simulink model "TV_2017old"  (R2016a)
settings: Solver=FixedStepAuto  StartTime=0.0  StopTime=inf  FixedStep=0.001  RelTol=1e-3
PreLoadFcn:
  | TV_2017_parameters
values from neighbouring files (symbols this model uses):
  battery_voltage = single(530)    [HIL_parameters.m]    (also in HIL_parameters_2018.m; TV_2017_parameters.m; TV_2017_parameters_VD.m)
  car_params = Simulink_Car_params    [HIL_parameters.m]    (also in HIL_parameters_2018.m; TV_2017_parameters.m; TV_2017_parameters_VD.m)
  i_Diff = 16    [HIL_parameters.m]    (also in HIL_parameters_2018.m; TV_2017_parameters.m)
  Kp = 1    [HIL_parameters.m]    (also in HIL_parameters_2018.m; TV_2017_parameters.m; TV_2017_parameters_VD.m)
  motor_data = struct    [HIL_parameters.m]    (also in HIL_parameters_2018.m; TV_2017_parameters.m)
  powerLimitControl = Simulink_el    [HIL_parameters.m]    (also in HIL_parameters_2018.m; TV_2017_parameters.m; TV_2017_parameters_VD.m)
  settings = Simulink_Settings    [HIL_parameters.m]    (also in HIL_parameters_2018.m; TV_2017_parameters.m; TV_2017_parameters_VD.m)
  SpdC_BCC = 0    [HIL_parameters.m]    (also in HIL_parameters_2018.m; TV_2017_parameters.m; TV_2017_parameters_VD.m)
  Speed_Neg_sat = -21    [HIL_parameters.m]    (also in HIL_parameters_2018.m; TV_2017_parameters.m; TV_2017_parameters_VD.m)
  Speed_Pos_sat = 21    [HIL_parameters.m]    (also in HIL_parameters_2018.m; TV_2017_parameters.m; TV_2017_parameters_VD.m)
  SteeringAngleFL = [-23.80 -22.65 -21.50 -20.34 -19.18 -18.03 -16.86 -15.70 -14.53 -13.35 -12.18 -10.99 -9.80 -8.61 -7.40 -6.19 -4.97 -3.75 -2.51 -1.26 0 1.27 2.56 3.85 5.17 6.50 7.84 9.21 10.59 12.00 13.42 14.88 16.36 17.87 19.41 20.99 22.61 24.26 25.97 27.73 29.54]    [CarSetupAnalysis2018.m]    (also in HIL_parameters_2018.m; TV_2017_parameters.m; TV_2017_parameters_VD.m = [-24.129 -22.950 -21.772 -20.593 -19.413 -18.232 -17.050 -15)
  SteeringAngleFR = [-29.54 -27.73 -25.97 -24.26 -22.61 -20.99 -19.41 -17.87 -16.36 -14.88 -13.42 -12.00 -10.59 -9.21 -7.84 -6.50 -5.17 -3.85 -2.56 -1.27 0 1.26 2.51 3.75 4.97 6.19 7.40 8.61 9.80 10.99 12.18 13.35 14.53 15.70 16.86 18.03 19.18 20.34 21.50 22.65 23.80]    [CarSetupAnalysis2018.m]    (also in HIL_parameters_2018.m; TV_2017_parameters.m; TV_2017_parameters_VD.m = [-29.3050 -27.5340 -25.8140 -24.1410 -22.5110 -20.9180 -19.3)
  SteeringWhAngle = [-105 -99.75 -94.5 -89.25 -84 -78.75 -73.5 -68.25 -63 -57.75 -52.5 -47.25 -42 -36.75 -31.5 -26.25 -21.0 -15.75 -10.5 -5.25 0.0 5.25 10.50 15.75 21.00 26.25 31.50 36.75 42.00 47.25 52.50 57.75  63.00 68.25 73.50 78.75 84.00 89.25 94.50 99.75 105.00]    [TV_2017_parameters_VD.m]
  Tn_n = 0    [HIL_parameters.m]    (also in HIL_parameters_2018.m; TV_2017_parameters.m; TV_2017_parameters_VD.m)
  tractionControl = Simulink_tc    [HIL_parameters.m]    (also in HIL_parameters_2018.m; IterativeTractionControlTuning.m; TV_2017_parameters.m; TV_2017_parameters_VD.m)
  yawRateControl = Simulink_yawRate    [HIL_parameters.m]    (also in HIL_parameters_2018.m; TV_2017_parameters.m; TV_2017_parameters_VD.m)
undefined symbols (not defined in the file or in its folder): DiscIntNeverNeededParam, magnitude, speedEstimation, TC_Decr_Gas, TC_Derivative, TC_Incr_Gas, TC_On, TC_Relay_Off, TC_Relay_On
libraries: CarMaker4SL x274, simulink_extras x45, simulink x37, dspfdesign x2
(part 2 of 14)

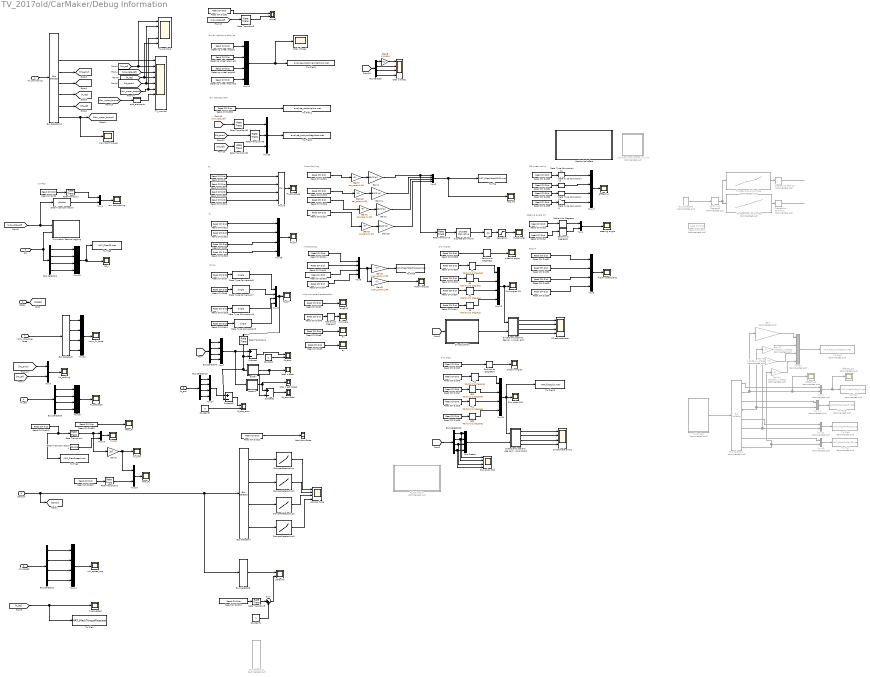
== system TV_2017old/CarMaker/Debug Information  ==
  note: SimRes
  note: Eff wheel radius
  note: motortorques
  note: Friction
  note: FZ CM
  note: Fy
  note: FX
  note: misc movement acceleration
  note: Steering angle CM
  note: Motor Rpm log
  note: Slip Angles
  note: Slip rates
  note: Yaw rate regulator
  note: Driver intentions analyze
  TV_monitoring : Inport
  states : Inport  Port=2
  whl_speed : Inport  Port=3
  Fx_est : Inport  Port=4
  "SR " : Inport  Port=5
  Sensors : Inport  Port=6
  norm_long_tire_force : Inport  Port=7
  Fz_acc : Inport  Port=8
  Abs : Abs
  "Aero downforce " : Scope
  Aero_Fx : Scope
  Aero_Fz : Scope
  Bus Creator : BusCreator  Inputs=4
  Bus Selector : BusSelector  OutputSignals=power,Input_throttle,Input_brake,KERS_pos
  Bus Selector1 : BusSelector  Commented=on  OutputSignals=Pm_FL,Pe_FL,Pm_FR,Pe_FR,Pm_RL,Pe_RL,Pm_RR,Pe_RR
  Bus Selector10 : BusSelector  OutputSignals=SR_FL,SR_FR,SR_RL,SR_RR
  Bus Selector11 : BusSelector  Commented=on  OutputSignals=steering_wheel_angle
  Bus Selector12 : BusSelector  OutputSignals=active_contraints,saturated_constraints,percentage_delivered_torque,Mz_error,yaw_rate_ref,T_req,Mz_ref,maxMotorTorque
  Bus Selector{2..5,13} (5 alike) : BusSelector  OutputSignals=FL,FR,RL,RR
  Bus Selector6 : BusSelector  OutputSignals=Fz_FL,Fz_FR,Fz_RL,Fz_RR
  Bus Selector7 : BusSelector  OutputSignals=damper_rate_FL,damper_rate_FR,damper_rate_RL,damper_rate_RR
  Bus Selector8 : BusSelector  OutputSignals=steering_wheel_angle
  Bus Selector9 : BusSelector  Commented=on  OutputSignals=steering_wheel_angle
  Constant : Constant  Value=0
  Constant1 : Constant
  Constant2 : Constant  Value=0
  DamperRateLookup : Lookup_n-D  NumberOfTableDimensions=1  BreakpointsForDimension1=car_params.damper_table_breakpoint;  Table=car_params.damper_pull_push_values_front;  ExtrapMethod=Clip  UseLastTableValue=on  InternalRulePriority=Speed  RndMeth=Simplest  InputSameDT=on
  DamperRateLookup1 : Lookup_n-D  NumberOfTableDimensions=1  BreakpointsForDimension1=car_params.damper_table_breakpoint;  Table=car_params.damper_pull_push_values_front;  ExtrapMethod=Clip  UseLastTableValue=on  InternalRulePriority=Speed  RndMeth=Simplest  InputSameDT=on
  DamperRateLookup2 : Lookup_n-D  NumberOfTableDimensions=1  BreakpointsForDimension1=car_params.damper_table_breakpoint;  Table=car_params.damper_pull_push_values_rear;  ExtrapMethod=Clip  UseLastTableValue=on  InternalRulePriority=Speed  RndMeth=Simplest  InputSameDT=on
  DamperRateLookup3 : Lookup_n-D  NumberOfTableDimensions=1  BreakpointsForDimension1=car_params.damper_table_breakpoint;  Table=car_params.damper_pull_push_values_rear;  ExtrapMethod=Clip  UseLastTableValue=on  InternalRulePriority=Speed  RndMeth=Simplest  InputSameDT=on
  Data Type Conversion : DataTypeConversion  OutDataTypeStr=double
  Data Type Conversion1 : DataTypeConversion  OutDataTypeStr=double
  Data Type Conversion{6..13} (8 alike) : DataTypeConversion  OutDataTypeStr=single
  Degrees to Radians : simulink_extras/Transformations/Degrees to Radians  Commented=on
  Degrees to Radians1 : simulink_extras/Transformations/Degrees to Radians  Commented=on
  Discrete Derivative : simulink/Discrete/Discrete Derivative  gainval=1.0  ICPrevScaledInput=0.0  InputProcessing=Inherited  OutMin=[]  OutMax=[]  OutDataType=fixdt(1, 16)  OutScaling=2^-10  DoSatur=off
  Extract and scale to deg compare to CM output in individual error : Subsystem
  Extract and scale to deg compare to CM output in individual error1 : Subsystem
  FL : simulink_extras/Transformations/Radians to Degrees
  FL steer ang lookup deg : Lookup_n-D  Commented=on  NumberOfTableDimensions=1  BreakpointsForDimension1=SteeringWhAngle  Table=SteeringAngleFL  ExtrapMethod=Clip  UseLastTableValue=on  InternalRulePriority=Speed  RndMeth=Simplest  InputSameDT=on
  FL1 : simulink_extras/Transformations/Radians to Degrees
  FR : simulink_extras/Transformations/Radians to Degrees
  FR steer ang lookup deg : Lookup_n-D  Commented=on  NumberOfTableDimensions=1  BreakpointsForDimension1=SteeringWhAngle  Table=SteeringAngleFR  ExtrapMethod=Clip  UseLastTableValue=on  InternalRulePriority=Speed  RndMeth=Simplest  InputSameDT=on
  FR1 : simulink_extras/Transformations/Radians to Degrees
  FY_CM : Scope
  Fl_derivate : Scope
  Fx_CM_scope : Scope
  Fx_estScope : Scope
  Fz_CM : Scope
  Fz_Estimation : Subsystem  Commented=on  TreatAsAtomicUnit=on
  Fz_acc_error : Scope  NumInputPorts=2
  Fz_error : Scope  NumInputPorts=2
  Fz_error total : Scope
  Gain{,12..14} (4 alike) : Gain  Commented=on  Gain=1/battery_voltage
  Gain{1,3,7,10} (4 alike) : Gain  Gain=car_params.GR
  Gain{2,4,11,15} (4 alike) : Gain  Gain=60/(2*pi)
  Gain5 : Gain  Gain=1/car_params.GR
  Gain6 : Gain  Gain=1/car_params.GR
  Gain8 : Gain  Gain=1/10000
  Gain9 : Gain  Gain=3.6
  Mechanical effect : Subsystem
  "Motor Torques " : Scope
  Mux{1,4,9..10,20} (5 alike) : Mux  Inputs=2
  Mux{5,11..13} (4 alike) : Mux  Commented=on  Inputs=2
  Mux{2..3,6..8,14..19,22..24,26..27} (16 alike) : Mux
  Mux21 : Mux  Commented=on
  Mux25 : Mux  Inputs=3
  Mz_tracking : Scope
  RL : simulink_extras/Transformations/Radians to Degrees
  RL1 : simulink_extras/Transformations/Radians to Degrees
  RR : simulink_extras/Transformations/Radians to Degrees
  RR1 : simulink_extras/Transformations/Radians to Degrees
  Radians to Degrees{,1..2,4,7} (5 alike) : simulink_extras/Transformations/Radians to Degrees
  Radians to Degrees3 : simulink_extras/Transformations/Radians to Degrees  Commented=on
  Rate Transition{,1..5} (6 alike) : RateTransition  OutPortSampleTime=matlab_params.control_system_sample_time
  Rate Transition{6,49..51} (4 alike) : RateTransition  OutPortSampleTimeOpt=Inherit
  Read CM Dict : CarMaker4SL/Read CM Dict  xname=Vhcl.FL.Fx  xsync=off
  Read CM Dict1 : CarMaker4SL/Read CM Dict  xname=Car.LongSlipRL  xsync=off
  Read CM Dict10 : CarMaker4SL/Read CM Dict  xname=Car.vx  xsync=off
  Read CM Dict11 : CarMaker4SL/Read CM Dict  xname=Vhcl.RR.Fz  xsync=off
  Read CM Dict12 : CarMaker4SL/Read CM Dict  xname=Car.Aero.Frc_1.z  xsync=off
  Read CM Dict13 : CarMaker4SL/Read CM Dict  xname=Vhcl.Steer.Ang  xsync=off
  Read CM Dict14 : CarMaker4SL/Read CM Dict  Commented=on  xsync=off
  Read CM Dict15 : CarMaker4SL/Read CM Dict  xname=Car.LongSlipRR  xsync=off
  Read CM Dict16 : CarMaker4SL/Read CM Dict  xname=Car.LongSlipRL  xsync=off
  Read CM Dict17 : CarMaker4SL/Read CM Dict  xname=Car.SlipAngleRR  xsync=off
  Read CM Dict18 : CarMaker4SL/Read CM Dict  xname=Vhcl.FR.Fx  xsync=off
  Read CM Dict19 : CarMaker4SL/Read CM Dict  xname=Vhcl.RR.Fx  xsync=off
  Read CM Dict2 : CarMaker4SL/Read CM Dict  xname=Car.YawRate  xsync=off
  Read CM Dict20 : CarMaker4SL/Read CM Dict  xname=Vhcl.RL.Fx  xsync=off
  Read CM Dict21 : CarMaker4SL/Read CM Dict  xname=Vhcl.FL.Fy  xsync=off
  Read CM Dict22 : CarMaker4SL/Read CM Dict  xname=Vhcl.FR.Fy  xsync=off
  Read CM Dict23 : CarMaker4SL/Read CM Dict  xname=Vhcl.RR.Fy  xsync=off
  Read CM Dict24 : CarMaker4SL/Read CM Dict  xname=Car.WheelSpd_FL  xsync=off
  Read CM Dict25 : CarMaker4SL/Read CM Dict  xname=Car.WheelSpd_FR  xsync=off
  Read CM Dict26 : CarMaker4SL/Read CM Dict  xname=Car.WheelSpd_RL  xsync=off
  Read CM Dict27 : CarMaker4SL/Read CM Dict  xname=Car.WheelSpd_RR  xsync=off
  Read CM Dict28 : CarMaker4SL/Read CM Dict  xname=Vhcl.RL.Fz  xsync=off
  Read CM Dict29 : CarMaker4SL/Read CM Dict  xname=Car.muRoadRL  xsync=off
  Read CM Dict3 : CarMaker4SL/Read CM Dict  xname=Car.CFR.rz  xsync=off
  Read CM Dict30 : CarMaker4SL/Read CM Dict  xname=Car.muRoadRR  xsync=off
  Read CM Dict31 : CarMaker4SL/Read CM Dict  xname=Car.muRoadFL  xsync=off
  Read CM Dict32 : CarMaker4SL/Read CM Dict  xname=Car.muRoadFR  xsync=off
  Read CM Dict33 : CarMaker4SL/Read CM Dict  xname=Car.WFL.Radius  xsync=off
  Read CM Dict34 : CarMaker4SL/Read CM Dict  xname=Car.WFR.Radius  xsync=off
  Read CM Dict35 : CarMaker4SL/Read CM Dict  xname=Car.WRR.Radius  xsync=off
  Read CM Dict36 : CarMaker4SL/Read CM Dict  xname=Car.WRL.Radius  xsync=off
  Read CM Dict37 : CarMaker4SL/Read CM Dict  xname=Car.SlipAngleRL  xsync=off
  Read CM Dict38 : CarMaker4SL/Read CM Dict  xname=Car.SideSlipAngle  xsync=off
  Read CM Dict39 : CarMaker4SL/Read CM Dict  xname=Car.SlipAngleFL  xsync=off
  Read CM Dict4 : CarMaker4SL/Read CM Dict  xname=Car.CFL.rz  xsync=off
  Read CM Dict40 : CarMaker4SL/Read CM Dict  xname=Car.SlipAngleFR  xsync=off
  Read CM Dict41 : CarMaker4SL/Read CM Dict  xname=PT.WFL.Trq_Drive  xsync=off
  Read CM Dict42 : CarMaker4SL/Read CM Dict  xname=PT.WFR.Trq_Drive  xsync=off
  Read CM Dict43 : CarMaker4SL/Read CM Dict  xname=PT.WRL.Trq_Drive  xsync=off
  Read CM Dict44 : CarMaker4SL/Read CM Dict  xname=PT.WRR.Trq_Drive  xsync=off
  Read CM Dict45 : CarMaker4SL/Read CM Dict  xname=Car.SideSlipAngle  xsync=off
  Read CM Dict46 : CarMaker4SL/Read CM Dict  xname=Car.LongSlipFL  xsync=off
  Read CM Dict47 : CarMaker4SL/Read CM Dict  xname=Car.LongSlipFR  xsync=off
  Read CM Dict48 : CarMaker4SL/Read CM Dict  xname=Vhcl.Roll  xsync=off
  Read CM Dict49 : CarMaker4SL/Read CM Dict  xname=Car.Aero.Frc_1.z  xsync=off
  Read CM Dict5 : CarMaker4SL/Read CM Dict  xname=Vhcl.RL.Fy  xsync=off
  Read CM Dict50 : CarMaker4SL/Read CM Dict  xname=Vhcl.YawRate  xsync=off
  Read CM Dict51 : CarMaker4SL/Read CM Dict  xname=Vhcl.YawRate  xsync=off
  Read CM Dict53 : CarMaker4SL/Read CM Dict  xname=Car.Aero.Frc_1.x  xsync=off
  Read CM Dict6 : CarMaker4SL/Read CM Dict  xname=Vhcl.FR.Fz  xsync=off
  Read CM Dict7 : CarMaker4SL/Read CM Dict  xname=Vhcl.FL.Fz  xsync=off
  Read CM Dict8 : CarMaker4SL/Read CM Dict  xname=Car.ax  xsync=off
  Read CM Dict9 : CarMaker4SL/Read CM Dict  xname=Car.ay  xsync=off
  SA calculation : Subsystem
  SA estimate error : Scope  NumInputPorts=4
  SA estimate error1 : Scope  NumInputPorts=4
  SR_i : Scope
  Saturation : Saturate  UpperLimit=50000
  Simulation Results Logging : Subsystem
  Slip angles CM : Scope
  Slip ratios CM1 : Scope
  Slip ratios CM2 : Scope  NumInputPorts=4
  Steering wheel ang-vel2 : CarMaker4SL/Read CM Dict  xname=DM.Steer.AngVel  xsync=off
  Steering wheel ang-vel3 : CarMaker4SL/Read CM Dict  xname=DM.Brake  xsync=off
  Steering wheel angle2 : CarMaker4SL/Read CM Dict  xname=DM.Steer.Ang  xsync=off
  Steering wheel angle3 : CarMaker4SL/Read CM Dict  xname=DM.Gas  xsync=off
  Subsystem : Subsystem  Commented=on
  Subtract : Sum  Inputs=+-
  Subtract1 : Sum  Inputs=+-
  Subtract2 : Sum  Inputs=+-
  Sum : Sum  Inputs=|++
  TV_monitor : Scope  NumInputPorts=9
  TV_monitor1 : Scope  NumInputPorts=5
  "T_requested " : Scope
  To File : ToFile  Filename=MAT_files\MotorRPMS.mat  MatrixName=MotorRpms  SaveFormat=Timeseries
  To File1 : ToFile  Filename=MAT_files\TorqueRequest  MatrixName=TorqueRequest  SaveFormat=Timeseries
  To File10 : ToFile  Filename=analyse_mat/yawRegulator.mat  MatrixName=yaw_reg  SaveFormat=Timeseries
  To File11 : ToFile  Filename=analyse_mat/trueYaw.mat  MatrixName=vhclYaw  SaveFormat=Timeseries
  To File12 : ToFile  Filename=analyse_mat/driverIntentions.mat  MatrixName=driverIntentions  SaveFormat=Timeseries
  To File13 : ToFile  Filename=MAT_files\slip.mat  MatrixName=slipratio  SaveFormat=Timeseries
  To File2 : ToFile  Filename=MAT_files\Speed.mat  MatrixName=VehicleSpeed  SaveFormat=Timeseries
  To File3 : ToFile  Filename=MAT_files\MotorTorques.mat  MatrixName=MotorTorques  SaveFormat=Timeseries
  To File4 : ToFile  Commented=on  Filename=MAT_files\PmPe_FL.mat  MatrixName=PmPe_FL  SaveFormat=Timeseries
  To File5 : ToFile  Commented=on  Filename=MAT_files\PmPe_FR.mat  MatrixName=PmPe_FR  SaveFormat=Timeseries
  To File6 : ToFile  Commented=on  Filename=MAT_files\PmPe_RL.mat  MatrixName=PmPe_RL  SaveFormat=Timeseries
  To File7 : ToFile  Commented=on  Filename=MAT_files\PmPe_RR.mat  MatrixName=PmPe_RR  SaveFormat=Timeseries
  To File8 : ToFile  Filename=MAT_files\SR.mat  MatrixName=SR  SaveFormat=Timeseries
  To File9 : ToFile  Commented=on  Filename=MAT_files\currentDraw.mat  SaveFormat=Timeseries
  Vehicle dynamics analysis JMH : Subsystem  Commented=on
  Vx_kmh : Scope
  "Vx_ms " : Scope
  Yaw rate tracking : Scope
  add_elements : Subsystem
  addall : Subsystem
  addall1 : Subsystem
  ax : Scope
  ay : Scope
  damper force : Scope  NumInputPorts=4
  delta SW : Scope  NumInputPorts=2
  effRadius : Scope
  effectFL_el : Scope  Commented=on
  effectFL_el1 : Scope  Commented=on
  eng rot : Scope
  friction coefficients : Scope
  "longSlip " : Scope
  maxMotorTorques : Scope
  norm_Fx_force : Scope
  rollAngle : Scope
  sideslip angle : Scope
  sideslip angle1 : Scope
  steering angle : Scope
  total z estimated : Scope
  total z force : Scope
  total z force1 : Scope
  total z force2 : Scope  NumInputPorts=4
  whl_speed_cog : Scope
  yawref : Scope  NumInputPorts=2
  wires:
  [T_req] -> To File1/1, "T_requested "/1
  [Mz_error] -> Mux9/1  "error"
  [Mz_ref] -> Mux9/2  "ref"
  Mux9/1 -> Mz_tracking/1
  Mux5/1 -> effectFL_el1/1, To File4/1
  Mux11/1 -> To File5/1
  Mux12/1 -> To File6/1
  Mux13/1 -> To File7/1
  Subsystem/1(Power debug) -> Bus Selector1/1
  Bus Selector1/1 -> Mux5/1  "<Pm_FL>"
  Bus Selector1/2 -> Gain/1, effectFL_el/1, Mux5/2  "<Pe_FL>"
  Bus Selector1/3 -> Mux11/1  "<Pm_FR>"
  Bus Selector1/4 -> Gain12/1, Mux11/2  "<Pe_FR>"
  Bus Selector1/5 -> Mux12/1  "<Pm_RL>"
  Bus Selector1/6 -> Gain13/1, Mux12/2  "<Pe_RL>"
  Bus Selector1/7 -> Mux13/1  "<Pm_RR>"
  Bus Selector1/8 -> Gain14/1, Mux13/2  "<Pe_RR>"
  whl_speed/1 -> Bus Selector2/1
  Bus Selector2/4 -> Mux14/4  "<RR>"
  Bus Selector2/3 -> Mux14/3  "<RL>"
  Bus Selector2/2 -> Mux14/2  "<FR>"
  Bus Selector2/1 -> Mux14/1  "<FL>"
  Mux14/1 -> whl_speed_cog/1
  Fx_est/1 -> Bus Selector3/1
  Bus Selector3/1 -> Mux15/1  "<FL>"
  Bus Selector3/2 -> Mux15/2  "<FR>"
  Bus Selector3/3 -> Mux15/3  "<RL>"
  Bus Selector3/4 -> Mux15/4  "<RR>"
  Mux15/1 -> Fx_estScope/1
  Read CM Dict53/1 -> Aero_Fx/1  "FL"
  Read CM Dict10/1 -> To File2/1, Rate Transition1/1  "V_x"
  Mux10/1 -> "Vx_ms "/1
  Rate Transition1/1 -> Gain9/1, Mux10/1  "V_x"
  Data Type Conversion1/1 -> Mux10/2  "V_est"
  Gain9/1 -> Mux20/1, Vx_kmh/1
  Mux20/1 -> Aero_Fz/1
  Read CM Dict49/1 -> Rate Transition2/1  "FL"
  Rate Transition2/1 -> Mux20/2
  Gain/1 -> Mux21/1  "Current FL"
  Gain12/1 -> Mux21/2  "Current FR"
  Gain13/1 -> Mux21/3  "Current RL"
  Gain14/1 -> Mux21/4  "Current RR"
  Mux21/1 -> To File9/1
  norm_long_tire_force/1 -> Bus Selector5/1
  Bus Selector5/1 -> Mux22/1  "<FL>"
  Bus Selector5/4 -> Mux22/4  "<RR>"
  Bus Selector5/3 -> Mux22/3  "<RL>"
  Bus Selector5/2 -> Mux22/2  "<FR>"
  Mux22/1 -> norm_Fx_force/1
  Rate Transition3/1 -> Discrete Derivative/1
  Saturation/1 -> Fl_derivate/1
  Abs/1 -> Saturation/1
  Discrete Derivative/1 -> Abs/1
  Mux2/1 -> eng rot/1, To File/1
  Read CM Dict27/1 -> Gain3/1
  Read CM Dict26/1 -> Gain1/1
  Gain15/1 -> Mux2/4  "Motor_RPM"
  Gain3/1 -> Gain15/1
  Gain2/1 -> Mux2/3  "Motor_RPM"
  Gain1/1 -> Gain2/1
  Gain11/1 -> Mux2/2  "Motor_RPM"
  Gain10/1 -> Gain11/1
  Read CM Dict25/1 -> Gain10/1
  Read CM Dict24/1 -> Gain7/1
  Gain4/1 -> Mux2/1, Rate Transition3/1  "Motor_RPM"
  Gain7/1 -> Gain4/1
  Radians to Degrees1/1 -> Mux4/2
  Mux4/1 -> steering angle/1
  Read CM Dict3/1 -> Radians to Degrees/1
  Read CM Dict4/1 -> Radians to Degrees1/1
  Radians to Degrees/1 -> Mux4/1
  Read CM Dict48/1 -> Radians to Degrees7/1
  Radians to Degrees7/1 -> rollAngle/1
  Read CM Dict9/1 -> ay/1
  Read CM Dict8/1 -> ax/1
  Read CM Dict1/1 -> "longSlip "/1
  Mux16/1 -> Fx_CM_scope/1
  Read CM Dict18/1 -> Mux16/2  "Fx_FR"
  Read CM Dict19/1 -> Mux16/4  "Fx_RR"
  Read CM Dict20/1 -> Mux16/3  "Fx_RL"
  Read CM Dict/1 -> Mux16/1  "Fx_FL"
  Mux18/1 -> FY_CM/1
  Read CM Dict22/1 -> Mux18/2  "Fy_FR"
  Read CM Dict5/1 -> Mux18/3  "Fy_RL"
  Read CM Dict23/1 -> Mux18/4  "Fy_RR"
  Read CM Dict21/1 -> Mux18/1  "Fy_FL"
  Data Type Conversion10/1 -> Mux3/3  "RL"
  Data Type Conversion7/1 -> Mux3/2  "FR"
  Mux3/1 -> Rate Transition4/1, Fz_CM/1
  Read CM Dict7/1 -> Data Type Conversion8/1
  Read CM Dict11/1 -> Data Type Conversion9/1
  Read CM Dict6/1 -> Data Type Conversion7/1
  Data Type Conversion9/1 -> Mux3/4  "RR"
  Read CM Dict28/1 -> Data Type Conversion10/1
  Data Type Conversion8/1 -> Mux3/1  "FL"
  Read CM Dict30/1 -> Mux6/4  "RR"
  Read CM Dict29/1 -> Mux6/3  "RL"
  Read CM Dict32/1 -> Mux6/2  "FR"
  Mux6/1 -> friction coefficients/1
  Read CM Dict31/1 -> Mux6/1  "FL"
  Gain6/1 -> To File3/1
  Gain5/1 -> "Motor Torques "/1
  Read CM Dict43/1 -> Mux8/3  "Mot_RL"
  Read CM Dict44/1 -> Mux8/4  "Mot_RR"
  Read CM Dict41/1 -> Mux8/1  "Mot_FL"
  Mux8/1 -> Gain6/1, Gain5/1
  Read CM Dict42/1 -> Mux8/2  "Mot_FR"
  Mux17/1 -> effRadius/1
  Data Type Conversion6/1 -> Mux17/4  "R_RR"
  Read CM Dict35/1 -> Data Type Conversion6/1
  Read CM Dict34/1 -> Data Type Conversion13/1
  Data Type Conversion13/1 -> Mux17/2  "R_FR"
  Data Type Conversion11/1 -> Mux17/3  "R_RL"
  Data Type Conversion12/1 -> Mux17/1  "R_FL"
  Read CM Dict36/1 -> Data Type Conversion11/1
  Read CM Dict33/1 -> Data Type Conversion12/1
  Read CM Dict38/1 -> Radians to Degrees2/1
  Radians to Degrees2/1 -> sideslip angle/1
  Mux23/1 -> Extract and scale to deg compare to CM output in individual error/1(SA_CM), Slip angles CM/1
  Read CM Dict40/1 -> FR/1  "FR"
  Read CM Dict39/1 -> FL/1  "FL"
  Read CM Dict17/1 -> RR/1  "RL"
  RR/1 -> Mux23/4
  Read CM Dict37/1 -> RL/1  "RL"
  RL/1 -> Mux23/3
  FR/1 -> Mux23/2
  FL/1 -> Mux23/1
  [yaw_rate_ref] -> Data Type Conversion/1, Simulation Results Logging/1(r_ref)  "r_ref"
  Bus Selector4/4 -> Mux19/4  "<RR>"
  Mux19/1 -> SR_i/1, To File8/1
  Bus Selector4/1 -> Mux19/1  "<FL>"
  Bus Selector4/2 -> Mux19/2  "<FR>"
  Bus Selector4/3 -> Mux19/3  "<RL>"
  "SR "/1 -> Simulation Results Logging/2(SR), Bus Selector4/1
  Data Type Conversion/1 -> Mux1/2  "r_ref"
  Rate Transition/1 -> Mux1/1  "r"
  Mux1/1 -> Yaw rate tracking/1
  Read CM Dict2/1 -> Rate Transition/1  "r"
  Subtract/1 -> Fz_error/1
  Bus Selector6/1 -> Mux7/1  "<Fz_FL>"
  Bus Selector6/2 -> Mux7/2  "<Fz_FR>"
  Bus Selector6/3 -> Mux7/3  "<Fz_RL>"
  Bus Selector6/4 -> Mux7/4  "<Fz_RR>"
  Mux7/1 -> addall1/1(In1), Subtract/1
  Rate Transition4/1 -> Subtract2/2, addall/1(In1), Subtract/2
  addall/1(Out1) -> Subtract1/2, total z force/1
  addall1/1(Out1) -> total z estimated/1, Subtract1/1
  Subtract1/1 -> Fz_error total/1
  Read CM Dict12/1 -> "Aero downforce "/1
  DamperRateLookup/1 -> damper force/1  "Fz_damp_FL"
  Bus Selector7/1 -> DamperRateLookup/1  "<damper_rate_FL>"
  Bus Selector7/2 -> DamperRateLookup1/1  "<damper_rate_FR>"
  Bus Selector7/3 -> DamperRateLookup2/1  "<damper_rate_RL>"
  Bus Selector7/4 -> DamperRateLookup3/1  "<damper_rate_RR>"
  DamperRateLookup1/1 -> damper force/2
  DamperRateLookup2/1 -> damper force/3
  DamperRateLookup3/1 -> damper force/4
  Sensors/1 -> [sensor], Bus Selector8/1, Bus Selector7/1  "V_est"
  Constant/1 -> Fz_error/2
  Bus Selector8/1 -> delta SW/1  "<steering_wheel_angle>"
  Read CM Dict13/1 -> Rate Transition5/1
  Rate Transition5/1 -> Sum/1
  Sum/1 -> delta SW/2
  Constant1/1 -> Sum/2
  [states] -> Bus Selector6/1
  states/1 -> [states]
  SA calculation/1(Out1) -> Extract and scale to deg compare to CM output in individual error/2(In1)
  [sensor] -> SA calculation/1(In1)
  Extract and scale to deg compare to CM output in individual error/1(FL) -> SA estimate error/1
  Extract and scale to deg compare to CM output in individual error/2(FR) -> SA estimate error/2
  Extract and scale to deg compare to CM output in individual error/3(RL) -> SA estimate error/3
  Extract and scale to deg compare to CM output in individual error/4(RR) -> SA estimate error/4
  Radians to Degrees3/1 -> FL steer ang lookup deg/1, FR steer ang lookup deg/1
  Degrees to Radians1/1 -> ?
  FR steer ang lookup deg/1 -> Degrees to Radians1/1
  Degrees to Radians/1 -> ?
  FL steer ang lookup deg/1 -> Degrees to Radians/1
  Bus Selector9/1 -> Radians to Degrees3/1  "<steering_wheel_angle>"
  Read CM Dict45/1 -> Radians to Degrees4/1
  Radians to Degrees4/1 -> sideslip angle1/1
  Mux24/1 -> Extract and scale to deg compare to CM output in individual error1/1(SA_CM), To File13/1, Slip ratios CM1/1
  Read CM Dict47/1 -> FR1/1  "FR"
  Read CM Dict46/1 -> FL1/1  "FL"
  Read CM Dict15/1 -> RR1/1  "RL"
  RR1/1 -> Mux24/4
  Read CM Dict16/1 -> RL1/1  "RL"
  RL1/1 -> Mux24/3
  FR1/1 -> Mux24/2
  FL1/1 -> Mux24/1
  Extract and scale to deg compare to CM output in individual error1/1(FL) -> SA estimate error1/1
  Extract and scale to deg compare to CM output in individual error1/2(FR) -> SA estimate error1/2
  Extract and scale to deg compare to CM output in individual error1/3(RL) -> SA estimate error1/3
  Extract and scale to deg compare to CM output in individual error1/4(RR) -> SA estimate error1/4
  Bus Selector10/1 -> Slip ratios CM2/1, Bus Creator/1  "<SR_FL>"
  Bus Selector10/2 -> Slip ratios CM2/2, Bus Creator/2  "<SR_FR>"
  Bus Selector10/3 -> Slip ratios CM2/3, Bus Creator/3  "<SR_RL>"
  Bus Selector10/4 -> Slip ratios CM2/4, Bus Creator/4  "<SR_RR>"
  [states] -> Bus Selector10/1
  Bus Creator/1 -> Extract and scale to deg compare to CM output in individual error1/2(In1)
  TV_monitoring/1 -> Bus Selector12/1
  Bus Selector12/3 -> TV_monitor/1  "<percentage_delivered_torque>"
  Bus Selector12/4 -> [Mz_error]  "<Mz_error>"
  Bus Selector12/5 -> [yaw_rate_ref]  "<yaw_rate_ref>"
  Bus Selector12/6 -> [T_req]  "<T_req>"
  Bus Selector12/7 -> [Mz_ref]  "<Mz_ref>"
  [Mz_ref] -> TV_monitor1/1, TV_monitor/2
  [yaw_rate_ref] -> TV_monitor/3
  [T_req] -> TV_monitor1/5, TV_monitor/4
  [Mz_error] -> TV_monitor1/2, TV_monitor/5
  Read CM Dict50/1 -> To File11/1
  Rate Transition50/1 -> Mux25/1
  Rate Transition49/1 -> Mux25/2
  Rate Transition51/1 -> Mux25/3
  [yaw_rate_ref] -> Rate Transition50/1
  [Mz_error] -> Rate Transition49/1
  [Mz_ref] -> Rate Transition51/1
  Mux25/1 -> To File10/1
  Steering wheel ang-vel2/1 -> Mux26/2
  Steering wheel angle3/1 -> Mux26/3
  Steering wheel ang-vel3/1 -> Mux26/4
  Steering wheel angle2/1 -> Mux26/1
  Mux26/1 -> total z force1/1, To File12/1
  Bus Selector12/8 -> maxMotorTorques/1, [Max_motor_torque]  "<maxMotorTorque>"
  [Max_motor_torque] -> TV_monitor1/4, TV_monitor/6
  [Max_motor_torque] -> add_elements/1(In1)
  add_elements/1(Out1) -> TV_monitor/7
  ? -> Bus Selector11/1
  [states] -> Bus Selector/1
  Bus Selector/1 -> Gain8/1  "<power>"
  Bus Selector/2 -> total z force2/2  "<Input_throttle>"
  Bus Selector/3 -> total z force2/3  "<Input_brake>"
  Bus Selector/4 -> total z force2/4  "<KERS_pos>"
  Gain8/1 -> total z force2/1
  Read CM Dict51/1 -> yawref/1
  [yaw_rate_ref] -> Rate Transition6/1
  Rate Transition6/1 -> yawref/2
  Constant2/1 -> Fz_acc_error/2
  Subtract2/1 -> Fz_acc_error/1
  Bus Selector13/1 -> Mux27/1  "<FL>"
  Bus Selector13/2 -> Mux27/2  "<FR>"
  Bus Selector13/3 -> Mux27/3  "<RL>"
  Bus Selector13/4 -> Mux27/4  "<RR>"
  Fz_acc/1 -> Bus Selector13/1
  Mux27/1 -> Subtract2/1

== system TV_2017old/CarMaker/DrivMan3 ==
  note: There's rarely a reason to override DrivMan signals.
      | Use the VehicleControl interface for this purpose.
  Sync_In : Inport
  Env.Misc : Inport  Port=2
  BusCreator : BusCreator  Inputs=17
  Demux : Demux  Outputs=17
  DrivMan : S-Function  FunctionName=CM_Sfun  Parameters='DrivMan'  SFunctionDeploymentMode=off  EnableBusSupport=off
  Sync_Out : Outport
  DrivMan.Out : Outport  Port=2
  wires:
  Demux/17 -> BusCreator/17  "DrivMan Steering Trq"
  Demux/16 -> BusCreator/16  "DrivMan Steering AngAcc"
  Demux/15 -> BusCreator/15  "DrivMan Steering AngVel"
  Demux/14 -> BusCreator/14  "DrivMan Steering Ang"
  Demux/13 -> BusCreator/13  "DrivMan Gas"
  Demux/12 -> BusCreator/12  "DrivMan Clutch"
  Demux/11 -> BusCreator/11  "DrivMan BrakePark"
  Demux/10 -> BusCreator/10  "DrivMan Brake"
  Demux/9 -> BusCreator/9  "DrivMan GearNo"
  Demux/8 -> BusCreator/8  "DrivMan SelectorCtrl"
  Demux/7 -> BusCreator/7  "DrivMan UserSignal4"
  Demux/6 -> BusCreator/6  "DrivMan UserSignal3"
  Demux/5 -> BusCreator/5  "DrivMan UserSignal2"
  Demux/4 -> BusCreator/4  "DrivMan UserSignal1"
  Demux/3 -> BusCreator/3  "DrivMan UserSignal0"
  Demux/2 -> BusCreator/2  "DrivMan Key"
  Demux/1 -> BusCreator/1  "DrivMan SST"
  Env.Misc/1 -> DrivMan/2
  Sync_In/1 -> DrivMan/1
  DrivMan/1 -> Sync_Out/1
  BusCreator/1 -> DrivMan.Out/1
  DrivMan/2 -> Demux/1

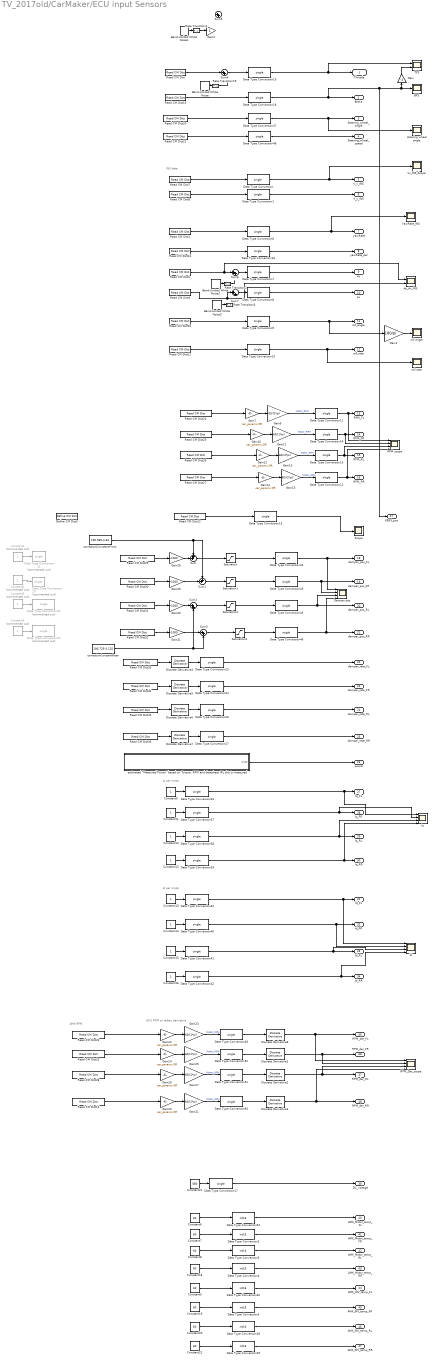
== system TV_2017old/CarMaker/ECU input Sensors  ==
  note: INS data
  note: ECU RPM to radian derivative
  note: AMK RPM
  note: Id per motor
  note: Iq per motor
  Ay_Ax_INS : Scope  NumInputPorts=2
  BPS : Scope
  Band-Limited White Noise : simulink/Sources/Band-Limited White Noise  Cov=[0.00002]  Ts=0.1  seed=[23341]
  Band-Limited White Noise1 : simulink/Sources/Band-Limited White Noise  Cov=[0.00002]  Ts=0.1  seed=[23341]
  Band-Limited White Noise2 : simulink/Sources/Band-Limited White Noise  Cov=[0.01]  Ts=0.1  seed=[23341]
  Band-Limited White Noise3 : simulink/Sources/Band-Limited White Noise  Cov=[0.01]  Ts=0.1  seed=[23341]
  Constant{1..4} (4 alike) : Constant  Commented=on
  Constant{9..16} (8 alike) : Constant
  Constant{5..8,18..20,22} (8 alike) : Constant  Value=60
  Constant21 : Constant  Value=580
  Damper pos : Scope  NumInputPorts=4
  Data Type Conversion{,1,6..19,24..27,32..33,37..52} (38 alike) : DataTypeConversion  OutDataTypeStr=single
  Data Type Conversion{2..5,28..30,54} (8 alike) : DataTypeConversion  OutDataTypeStr=int16
  Data Type Conversion{20..23} (4 alike) : DataTypeConversion  Commented=on  OutDataTypeStr=single
  Define CM Dict3 : CarMaker4SL/Define CM Dict  xname=KERS_pos  xmono=off  xtype=Double  xdvaplace=None  xnstates=0  xfirststate=0  xinitial=0
  Discrete Derivative{1..3,8} (4 alike) : simulink/Discrete/Discrete Derivative  gainval=1.0  ICPrevScaledInput=0.0  InputProcessing=Inherited  OutMin=[]  OutMax=[]  OutDataType=fixdt(1, 16)  OutScaling=2^-10  DoSatur=off
  Discrete Derivative{4..7} (4 alike) : simulink/Discrete/Discrete Derivative  gainval=1.0  ICPrevScaledInput=0.0  OutMin=[]  OutMax=[]  OutDataType=fixdt(1, 16)  OutScaling=2^-10  DoSatur=off
  Gain : Gain  Gain=-1
  Gain1 : Gain  Gain=180/pi
  Gain{7,10,12,14,20,22,24,26} (8 alike) : Gain  Gain=car_params.GR
  Gain{9,11,13,15,21,23,25,27} (8 alike) : Gain  Gain=60/(2*pi)
  Gain2 : Gain
  Gain{28..31} (4 alike) : Gain  Gain=-1000
  Id : Scope  NumInputPorts=4
  Iq : Scope  NumInputPorts=4
  RPM scope : Scope  NumInputPorts=4
  "RPM_Der_scope " : Scope  NumInputPorts=4
  Rate Transition{1..3,19} (4 alike) : RateTransition  OutPortSampleTimeOpt=Inherit  OutPortSampleTime=matlab_params.sensor_sampling_time
  Read CM Dict : CarMaker4SL/Read CM Dict  xname=VC.Gas  xsync=off
  Read CM Dict1 : CarMaker4SL/Read CM Dict  xname=Vhcl.YawRate  xsync=off
  Read CM Dict10 : CarMaker4SL/Read CM Dict  xname=Vhcl.Roll  xsync=off
  Read CM Dict11 : CarMaker4SL/Read CM Dict  xname=Vhcl.RollVel  xsync=off
  Read CM Dict12 : CarMaker4SL/Read CM Dict  xname=KERS_pos  xsync=off
  Read CM Dict13 : CarMaker4SL/Read CM Dict  xname=Vhcl.YawAcc  xsync=off
  Read CM Dict14 : CarMaker4SL/Read CM Dict  xname=Car.WheelSpd_RR  xsync=off
  Read CM Dict15 : CarMaker4SL/Read CM Dict  xname=VC.Brake  xsync=off
  Read CM Dict2 : CarMaker4SL/Read CM Dict  xname=Car.ay  xsync=off
  Read CM Dict20 : CarMaker4SL/Read CM Dict  xname=Vhcl.Steer.Ang  xsync=off
  Read CM Dict21 : CarMaker4SL/Read CM Dict  xname=Vhcl.Steer.Vel  xsync=off
  Read CM Dict22 : CarMaker4SL/Read CM Dict  xname=Car.WheelSpd_FL  xsync=off
  Read CM Dict23 : CarMaker4SL/Read CM Dict  xname=Car.WheelSpd_FR  xsync=off
  Read CM Dict24 : CarMaker4SL/Read CM Dict  xname=Car.WheelSpd_FL  xsync=off
  Read CM Dict25 : CarMaker4SL/Read CM Dict  xname=Car.WheelSpd_FR  xsync=off
  Read CM Dict26 : CarMaker4SL/Read CM Dict  xname=Car.WheelSpd_RL  xsync=off
  Read CM Dict27 : CarMaker4SL/Read CM Dict  xname=Car.WheelSpd_RR  xsync=off
  Read CM Dict28 : CarMaker4SL/Read CM Dict  xname=Car.WheelSpd_RL  xsync=off
  Read CM Dict29 : CarMaker4SL/Read CM Dict  xname=Car.SpringFL.l  xsync=off
  Read CM Dict30 : CarMaker4SL/Read CM Dict  xname=Car.SpringFR.l  xsync=off
  Read CM Dict31 : CarMaker4SL/Read CM Dict  xname=Car.SpringRL.l  xsync=off
  Read CM Dict32 : CarMaker4SL/Read CM Dict  xname=Car.SpringRR.l  xsync=off
  Read CM Dict33 : CarMaker4SL/Read CM Dict  xname=Car.SpringFL.l  xsync=off
  Read CM Dict34 : CarMaker4SL/Read CM Dict  xname=Car.SpringFR.l  xsync=off
  Read CM Dict35 : CarMaker4SL/Read CM Dict  xname=Car.SpringRL.l  xsync=off
  Read CM Dict36 : CarMaker4SL/Read CM Dict  xname=Car.SpringRR.l  xsync=off
  Read CM Dict7 : CarMaker4SL/Read CM Dict  xname=Car.vx  xsync=off
  Read CM Dict8 : CarMaker4SL/Read CM Dict  xname=Car.vy  xsync=off
  Read CM Dict9 : CarMaker4SL/Read CM Dict  xname=Car.ax  xsync=off
  Saturation{,1..3} (4 alike) : Saturate  UpperLimit=200  LowerLimit=0.001
  Scope : Scope
  Sum : Sum  Inputs=++|
  Sum1 : Sum  Inputs=++|
  Sum{2..7} (6 alike) : Sum  Inputs=|++
  TPS : Scope  NumInputPorts=2
  Vx_INS_Scope : Scope
  YawRate_INS : Scope
  correctionConstantRear : Constant  Value=190.725-3.125
  correctionCornstantFront : Constant  Value=190.965-3.63
  "estimated \"Measured Power\" based on Torque, RPM and datasheet IRL this is measured" : Subsystem
  "roll angle " : Scope
  roll rate : Scope
  steering wheel angle : Scope
  "Throttle " : Outport
  "Brake " : Outport  Port=2
  "Steering_wheel_angle " : Outport  Port=3
  Steering_wheel_speed : Outport  Port=4
  V_x_INS : Outport  Port=5
  V_y_INS : Outport  Port=6
  yawRate : Outport  Port=7
  yawRate_der : Outport  Port=8
  ay : Outport  Port=9
  "ax " : Outport  Port=10
  roll_angle : Outport  Port=11
  roll_rate : Outport  Port=12
  RPM_FL : Outport  Port=13
  RPM_FR : Outport  Port=14
  RPM_RL : Outport  Port=15
  RPM_RR : Outport  Port=16
  KERS_pos : Outport  Port=17
  damper_pos_FL : Outport  Port=18
  damper_pos_FR : Outport  Port=19
  damper_pos_RL : Outport  Port=20
  damper_pos_RR : Outport  Port=21
  damper_rate_FL : Outport  Port=22
  damper_rate_FR : Outport  Port=23
  damper_rate_RL : Outport  Port=24
  damper_rate_RR : Outport  Port=25
  power : Outport  Port=26
  Iq_FL : Outport  Port=27
  Iq_FR : Outport  Port=28
  Iq_RL : Outport  Port=29
  Iq_RR : Outport  Port=30
  Id_FL : Outport  Port=31
  Id_FR : Outport  Port=32
  Id_RL : Outport  Port=33
  Id_RR : Outport  Port=34
  RPM_der_FL : Outport  Port=35
  RPM_der_FR : Outport  Port=36
  RPM_der_RL : Outport  Port=37
  RPM_der_RR : Outport  Port=38
  DC_voltage : Outport  Port=39
  AMK_Motor_temp_FL : Outport  Port=40
  AMK_Motor_temp_FR : Outport  Port=41
  AMK_Motor_temp_RL : Outport  Port=42
  AMK_Motor_temp_RR : Outport  Port=43
  AMK_INV_temp_FL : Outport  Port=44
  AMK_INV_temp_FR : Outport  Port=45
  AMK_INV_temp_RL : Outport  Port=46
  AMK_INV_temp_RR : Outport  Port=47
  wires:
  Gain7/1 -> Gain9/1
  Read CM Dict24/1 -> Gain7/1
  Read CM Dict25/1 -> Gain10/1
  Gain10/1 -> Gain11/1
  Gain12/1 -> Gain13/1
  Gain14/1 -> Gain15/1
  Read CM Dict26/1 -> Gain12/1
  Read CM Dict27/1 -> Gain14/1
  Gain9/1 -> Data Type Conversion11/1  "Motor_RPM"
  Gain15/1 -> Data Type Conversion12/1  "Motor_RPM"
  Gain13/1 -> Data Type Conversion13/1  "Motor_RPM"
  Gain11/1 -> Data Type Conversion14/1  "Motor_RPM"
  Data Type Conversion11/1 -> RPM scope/1, RPM_FL/1
  Data Type Conversion14/1 -> RPM scope/2, RPM_FR/1
  Data Type Conversion13/1 -> RPM scope/3, RPM_RL/1
  Data Type Conversion12/1 -> RPM scope/4, RPM_RR/1
  Read CM Dict12/1 -> Data Type Conversion15/1
  Data Type Conversion15/1 -> Scope/1
  Read CM Dict15/1 -> Data Type Conversion18/1
  Data Type Conversion18/1 -> KERS_pos/1, BPS/1, Gain/1, "Brake "/1
  Data Type Conversion19/1 -> TPS/1, "Throttle "/1
  Constant1/1 -> Data Type Conversion21/1
  Constant2/1 -> Data Type Conversion20/1
  Constant3/1 -> Data Type Conversion22/1
  Constant4/1 -> Data Type Conversion23/1
  Data Type Conversion25/1 -> damper_rate_FL/1
  Discrete Derivative4/1 -> Data Type Conversion25/1
  Data Type Conversion24/1 -> damper_rate_FR/1
  Discrete Derivative5/1 -> Data Type Conversion24/1
  Data Type Conversion26/1 -> damper_rate_RL/1
  Discrete Derivative6/1 -> Data Type Conversion26/1
  Data Type Conversion27/1 -> damper_rate_RR/1
  Discrete Derivative7/1 -> Data Type Conversion27/1
  Read CM Dict20/1 -> Data Type Conversion47/1
  Read CM Dict21/1 -> Data Type Conversion48/1
  Data Type Conversion47/1 -> steering wheel angle/1, "Steering_wheel_angle "/1
  Data Type Conversion48/1 -> Steering_wheel_speed/1
  Data Type Conversion17/1 -> DC_voltage/1
  Constant21/1 -> Data Type Conversion17/1
  Read CM Dict30/1 -> Gain29/1
  Read CM Dict31/1 -> Gain30/1
  Read CM Dict32/1 -> Gain31/1
  Read CM Dict29/1 -> Gain28/1
  Data Type Conversion43/1 -> Damper pos/2, damper_pos_FR/1
  Data Type Conversion45/1 -> Damper pos/3, damper_pos_RL/1
  Data Type Conversion44/1 -> Damper pos/1, damper_pos_FL/1
  Data Type Conversion46/1 -> Damper pos/4, damper_pos_RR/1
  Sum/1 -> Saturation/1
  Gain30/1 -> Sum2/1
  Gain31/1 -> Sum3/1
  correctionConstantRear/1 -> Sum3/2, Sum2/2
  Sum1/1 -> Saturation1/1
  Sum2/1 -> Saturation2/1
  Sum3/1 -> Saturation3/1
  Saturation/1 -> Data Type Conversion44/1
  Saturation1/1 -> Data Type Conversion43/1
  Saturation2/1 -> Data Type Conversion45/1
  Saturation3/1 -> Data Type Conversion46/1
  Read CM Dict33/1 -> Discrete Derivative4/1
  Read CM Dict34/1 -> Discrete Derivative5/1
  Read CM Dict35/1 -> Discrete Derivative6/1
  Read CM Dict36/1 -> Discrete Derivative7/1
  Data Type Conversion30/1 -> AMK_INV_temp_FL/1
  Constant5/1 -> Data Type Conversion30/1
  Data Type Conversion54/1 -> AMK_Motor_temp_FL/1
  Constant6/1 -> Data Type Conversion54/1
  Data Type Conversion2/1 -> AMK_Motor_temp_FR/1
  Constant7/1 -> Data Type Conversion2/1
  Data Type Conversion3/1 -> AMK_Motor_temp_RL/1
  Constant8/1 -> Data Type Conversion3/1
  Data Type Conversion4/1 -> AMK_Motor_temp_RR/1
  Constant18/1 -> Data Type Conversion4/1
  Data Type Conversion5/1 -> AMK_INV_temp_FR/1
  Constant19/1 -> Data Type Conversion5/1
  Data Type Conversion28/1 -> AMK_INV_temp_RL/1
  Constant20/1 -> Data Type Conversion28/1
  Data Type Conversion29/1 -> AMK_INV_temp_RR/1
  Constant22/1 -> Data Type Conversion29/1
  Data Type Conversion33/1 -> Iq/1, Iq_FL/1
  Data Type Conversion37/1 -> Iq/2, Iq_FR/1
  Data Type Conversion38/1 -> Iq/3, Iq_RL/1
  Data Type Conversion39/1 -> Iq/4, Iq_RR/1
  Constant11/1 -> Data Type Conversion37/1
  Constant12/1 -> Data Type Conversion38/1
  Constant13/1 -> Data Type Conversion39/1
  Constant9/1 -> Data Type Conversion33/1
  Data Type Conversion32/1 -> Id/1, Id_FL/1
  Data Type Conversion40/1 -> Id/2, Id_FR/1
  Data Type Conversion41/1 -> Id/3, Id_RL/1
  Data Type Conversion42/1 -> Id/4, Id_RR/1
  Constant16/1 -> Data Type Conversion42/1
  Constant14/1 -> Data Type Conversion40/1
  Constant15/1 -> Data Type Conversion41/1
  Constant10/1 -> Data Type Conversion32/1
  Discrete Derivative1/1 -> "RPM_Der_scope "/2, RPM_der_FR/1
  Discrete Derivative2/1 -> "RPM_Der_scope "/3, RPM_der_RL/1
  Discrete Derivative3/1 -> "RPM_Der_scope "/4, RPM_der_RR/1
  Gain21/1 -> Data Type Conversion50/1  "Motor_RPM"
  Gain23/1 -> Data Type Conversion49/1  "Motor_RPM"
  Gain26/1 -> Gain27/1
  Gain25/1 -> Data Type Conversion52/1  "Motor_RPM"
  Data Type Conversion51/1 -> Discrete Derivative2/1
  Gain27/1 -> Data Type Conversion51/1  "Motor_RPM"
  Data Type Conversion52/1 -> Discrete Derivative1/1
  Data Type Conversion50/1 -> Discrete Derivative3/1
  Gain20/1 -> Gain21/1
  Gain24/1 -> Gain25/1
  Gain22/1 -> Gain23/1
  Read CM Dict22/1 -> Gain22/1
  Read CM Dict28/1 -> Gain26/1
  Read CM Dict14/1 -> Gain20/1
  Read CM Dict23/1 -> Gain24/1
  Data Type Conversion10/1 -> roll rate/1, roll_rate/1
  Data Type Conversion9/1 -> Gain1/1, roll_angle/1
  Data Type Conversion/1 -> V_x_INS/1, Vx_INS_Scope/1
  Data Type Conversion1/1 -> V_y_INS/1
  Data Type Conversion6/1 -> yawRate/1, YawRate_INS/1
  Data Type Conversion16/1 -> yawRate_der/1
  Data Type Conversion7/1 -> ay/1
  Data Type Conversion8/1 -> "ax "/1
  Read CM Dict2/1 -> Ay_Ax_INS/1, Sum6/1
  Read CM Dict9/1 -> Sum7/1, Ay_Ax_INS/2
  Read CM Dict13/1 -> Data Type Conversion16/1
  Read CM Dict11/1 -> Data Type Conversion10/1
  Read CM Dict10/1 -> Data Type Conversion9/1
  Read CM Dict8/1 -> Data Type Conversion1/1
  Read CM Dict7/1 -> Data Type Conversion/1
  Read CM Dict1/1 -> Data Type Conversion6/1
  "estimated \"Measured Power\" based on Torque, RPM and datasheet IRL this is measured"/1(Out2) -> power/1
  Gain1/1 -> "roll angle "/1
  Gain28/1 -> Sum/2
  Gain29/1 -> Sum1/2
  correctionCornstantFront/1 -> Sum/1, Sum1/1
  Gain/1 -> TPS/2
  Band-Limited White Noise/1 -> Rate Transition19/1
  Rate Transition19/1 -> ?
  Sum4/1 -> Data Type Conversion19/1
  Read CM Dict/1 -> Sum4/1
  Band-Limited White Noise1/1 -> Rate Transition1/1
  Band-Limited White Noise2/1 -> Rate Transition2/1
  Sum6/1 -> Data Type Conversion7/1
  Band-Limited White Noise3/1 -> Rate Transition3/1
  Sum7/1 -> Data Type Conversion8/1
  Rate Transition1/1 -> Gain2/1
  Rate Transition2/1 -> ?
  Data Type Conversion49/1 -> Discrete Derivative8/1
  Discrete Derivative8/1 -> "RPM_Der_scope "/1, RPM_der_FL/1

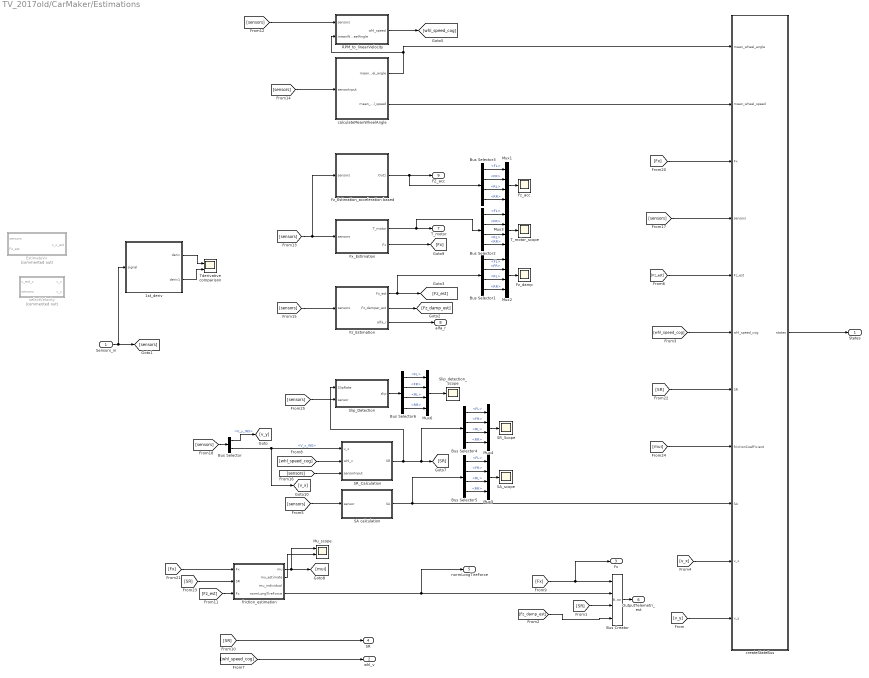
== system TV_2017old/CarMaker/Estimations ==
  Sensors_in : Inport
  1st_deriv : Subsystem
  Bus Creator : BusCreator  Inputs=4  OutDataTypeStr=Bus: OutputTelemetri_est
      settings: InheritFromInputs=off
  Bus Selector : BusSelector  OutputSignals=V_y_INS,V_x_INS
  Bus Selector{1..6} (6 alike) : BusSelector  OutputSignals=FL,FR,RL,RR
  EstimateVx : Subsystem  Commented=on
  Fx_Estimation : Subsystem
  Fz_Estimation : Subsystem  TreatAsAtomicUnit=on
  Fz_Estimation_acceleration based : Subsystem  TreatAsAtomicUnit=on
  Fz_acc : Scope
  Fz_damp : Scope
  Mu_scope : Scope  NumInputPorts=2
  Mux{1..6} (6 alike) : Mux
  RPM_to_linearVelocity : Subsystem
  SA calculation : Subsystem
  SA_scope : Scope
  SR_Calculation : Subsystem
  SR_Scope : Scope
  Slip_Detection : Subsystem
  Slip_detection_Scope : Scope
  T_motor_scope : Scope
  Tderivative comparison : Scope  NumInputPorts=2
  calculateMeanWheelAngle : Subsystem
  createStateBus : Subsystem
  friction_estimation : Subsystem
  selectVelocity : Subsystem  Commented=on
  States : Outport
  whl_v : Outport  Port=2
  Fx : Outport  Port=3
  SR : Outport  Port=4
  normLongTireForce : Outport  Port=5
  OutputTelemetri_est : Outport  Port=6
  T_motor : Outport  Port=7
  alfa_r : Outport  Port=8
  FZ_acc : Outport  Port=9
  wires:
  Fx_Estimation/2(Fx) -> [Fx]
  RPM_to_linearVelocity/1(whl_speed) -> [whl_speed_cog]
  createStateBus/1(states) -> States/1
  [v_y] -> createStateBus/11(v_y)
  [v_x] -> createStateBus/10(v_x)
  [whl_speed_cog] -> createStateBus/6(whl_speed_cog)
  Fz_Estimation/1(Fz_est) -> [Fz_est], Bus Selector1/1
  friction_estimation/1(mu) -> [mui], Mu_scope/1
  [whl_speed_cog] -> whl_v/1
  [Fx] -> Bus Creator/1, Fx/1
  [SR] -> SR/1
  friction_estimation/4(normLongTireForce) -> normLongTireForce/1, Bus Creator/2
  Bus Creator/1 -> OutputTelemetri_est/1
  [Fz_est] -> friction_estimation/3(Fz)
  calculateMeanWheelAngle/1(mean_wheel_angle) -> createStateBus/1(mean_wheel_angle), RPM_to_linearVelocity/2(meanWheelAngle)
  calculateMeanWheelAngle/2(mean_wheel_speed) -> createStateBus/2(mean_wheel_speed)
  Fx_Estimation/1(T_motor) -> Bus Selector2/1, T_motor/1
  [whl_speed_cog] -> SR_Calculation/2(whl_v)
  Sensors_in/1 -> 1st_deriv/1(signal), [sensors]
  [sensors] -> RPM_to_linearVelocity/1(sensors)
  [sensors] -> Fz_Estimation_acceleration based/1(sensors), Fx_Estimation/1(sensors)
  [sensors] -> calculateMeanWheelAngle/1(sensorInput)
  [sensors] -> Fz_Estimation/1(sensors)
  [sensors] -> SR_Calculation/3(sensorInput)
  [sensors] -> createStateBus/4(sensors)
  [sensors] -> Bus Selector/1
  Bus Selector/2 -> [v_x], SR_Calculation/1(v_x)  "<V_x_INS>"
  Bus Selector/1 -> [v_y]  "<V_y_INS>"
  [SR] -> Bus Creator/3
  Fz_Estimation/2(Fz_damper_est) -> [Fz_damp_est]
  [Fz_damp_est] -> Bus Creator/4
  Fz_Estimation/3(alfa_r) -> alfa_r/1
  [sensors] -> SA calculation/1(sensor)
  SA calculation/1(SA) -> Bus Selector5/1, createStateBus/9(SA)
  [Fz_est] -> createStateBus/5(Fz_est)
  [Fx] -> createStateBus/3(Fx)
  [Fx] -> friction_estimation/1(Fx)
  [SR] -> createStateBus/7(SR)
  [SR] -> friction_estimation/2(SR)
  [mui] -> createStateBus/8(frictionCoefficient)
  SR_Calculation/1(SR) -> Slip_Detection/1(SlipRate), Bus Selector4/1, [SR]
  [sensors] -> Slip_Detection/2(sensor)
  Fz_Estimation_acceleration based/1(Out1) -> Bus Selector3/1, FZ_acc/1
  Bus Selector3/1 -> Mux1/1  "<FL>"
  Bus Selector3/2 -> Mux1/2  "<FR>"
  Bus Selector3/3 -> Mux1/3  "<RL>"
  Bus Selector3/4 -> Mux1/4  "<RR>"
  Mux1/1 -> Fz_acc/1
  Bus Selector1/1 -> Mux2/1  "<FL>"
  Bus Selector1/2 -> Mux2/2  "<FR>"
  Bus Selector1/3 -> Mux2/3  "<RL>"
  Bus Selector1/4 -> Mux2/4  "<RR>"
  Mux2/1 -> Fz_damp/1
  Bus Selector2/1 -> Mux3/1  "<FL>"
  Bus Selector2/2 -> Mux3/2  "<FR>"
  Bus Selector2/3 -> Mux3/3  "<RL>"
  Bus Selector2/4 -> Mux3/4  "<RR>"
  Mux3/1 -> T_motor_scope/1
  Bus Selector4/1 -> Mux4/1  "<FL>"
  Bus Selector4/2 -> Mux4/2  "<FR>"
  Bus Selector4/3 -> Mux4/3  "<RL>"
  Bus Selector4/4 -> Mux4/4  "<RR>"
  Mux4/1 -> SR_Scope/1
  1st_deriv/1(deriv) -> Tderivative comparison/1
  1st_deriv/2(deriv1) -> Tderivative comparison/2
  friction_estimation/2(mu_estimate) -> Mu_scope/2
  Bus Selector5/1 -> Mux5/1  "<FL>"
  Bus Selector5/2 -> Mux5/2  "<FR>"
  Bus Selector5/3 -> Mux5/3  "<RL>"
  Bus Selector5/4 -> Mux5/4  "<RR>"
  Mux5/1 -> SA_scope/1
  Bus Selector6/1 -> Mux6/1  "<FL>"
  Bus Selector6/2 -> Mux6/2  "<FR>"
  Bus Selector6/3 -> Mux6/3  "<RL>"
  Bus Selector6/4 -> Mux6/4  "<RR>"
  Mux6/1 -> Slip_detection_Scope/1
  Slip_Detection/1(slip) -> Bus Selector6/1

== system TV_2017old/CarMaker/IPG Vehicle3 ==
  Sync_In : Inport
  Vhcl.Model.Source : Inport  Port=2
  VhclCtrl.Steering : Inport  Port=3
  Vhcl.Wheel.In : Inport  Port=4
  Vhcl.Misc : Inport  Port=5
  VhclCtrl.Brake : Inport  Port=6
  VhclCtrl.PT : Inport  Port=7
  Brake : Subsystem
  CarAndTrailer : Subsystem
  PowerTrain : Subsystem
  Stop Simulation : Stop
  VehicleSource_BuiltIn : simulink/Logic and Bit Operations/Compare To Constant  relop=~=  const=1  OutDataTypeStr=boolean  ZeroCross=off
  Sync_Out : Outport
  wires:
  VhclCtrl.PT/1 -> PowerTrain/3(VhclCtrl.PT)
  Brake/1(Sync_Out) -> PowerTrain/1(Sync_In)
  CarAndTrailer/1(Sync_Out) -> Brake/1(Sync_In)
  CarAndTrailer/2(Brake.IF.In) -> Brake/2(Brake.IF.In)
  VhclCtrl.Brake/1 -> Brake/3(VhclCtrl.Brake)
  PowerTrain/1(Sync_Out) -> Sync_Out/1
  Vhcl.Misc/1 -> CarAndTrailer/4(Vhcl.Misc)
  Vhcl.Wheel.In/1 -> CarAndTrailer/3(Vhcl.Wheel.In)
  VhclCtrl.Steering/1 -> CarAndTrailer/2(VhclCtrl.Steering)
  Sync_In/1 -> CarAndTrailer/1(Sync_In)
  Vhcl.Model.Source/1 -> VehicleSource_BuiltIn/1
  VehicleSource_BuiltIn/1 -> Stop Simulation/1
  Brake/2(Vhcl.Wheel.PT) -> PowerTrain/2(Vhcl.Wheel.PT)

== system TV_2017old/CarMaker/Open GUI ==
  S-Function : S-Function  FunctionName=cm_gui  SFunctionDeploymentMode=off  EnableBusSupport=off

== system TV_2017old/CarMaker/VehicleControl3 ==
  note: <Your model here>
  note: When implementing a vehicle control model,
      | be sure to add '-disablevehiclecontrol' to the command line arguments
      | in the CarMaker Model Configuration block.
      | Otherwise your model will possibly not see the original DrivMan signals
      | on its inputs, but those of a currently activated C-coded vehicle control model instead.
  Sync_In : Inport
  DrivMan.In : Inport  Port=2
  Bus Creator2 : BusCreator  Inputs=2
  CreateBus Vhcl.Misc : Subsystem
  CreateBus Vhcl.Wheel.In : Subsystem
  CreateBus VhclCtrl : Subsystem
  CreateBus VhclCtrl.PT : Subsystem
  CreateBus VhclCtrl.Steering : Subsystem
  Demux2 : Demux  Outputs=2
  VehicleControl : S-Function  FunctionName=CM_Sfun  Parameters='VehicleControl'  SFunctionDeploymentMode=off  EnableBusSupport=off
  VehicleControlUpd : S-Function  FunctionName=CM_Sfun  Parameters='VehicleControlUpd'  SFunctionDeploymentMode=off  EnableBusSupport=off
  Sync_Out : Outport
  Vhcl.Model.Source : Outport  Port=2
  VhclCtrl.Steering : Outport  Port=3
  Vhcl.Wheel.In : Outport  Port=4
  Vhcl.Misc : Outport  Port=5
  VhclCtrl.Brake : Outport  Port=6
  VhclCtrl.PT : Outport  Port=7
  wires:
  CreateBus VhclCtrl/1(Out) -> VehicleControlUpd/2
  VehicleControl/2 -> CreateBus VhclCtrl/1(In)
  VehicleControlUpd/2 -> Vhcl.Model.Source/1
  VehicleControlUpd/4 -> CreateBus Vhcl.Wheel.In/1(In1)
  VehicleControlUpd/5 -> CreateBus Vhcl.Misc/1(In1)
  VehicleControlUpd/6 -> Demux2/1
  VehicleControlUpd/7 -> CreateBus VhclCtrl.PT/1(In1)
  VehicleControlUpd/3 -> CreateBus VhclCtrl.Steering/1(In1)
  CreateBus Vhcl.Misc/1(Out1) -> Vhcl.Misc/1
  CreateBus Vhcl.Wheel.In/1(Out1) -> Vhcl.Wheel.In/1
  DrivMan.In/1 -> VehicleControl/2
  VehicleControl/1 -> VehicleControlUpd/1
  Sync_In/1 -> VehicleControl/1
  CreateBus VhclCtrl.PT/1(Out1) -> VhclCtrl.PT/1
  Bus Creator2/1 -> VhclCtrl.Brake/1
  CreateBus VhclCtrl.Steering/1(Out1) -> VhclCtrl.Steering/1
  VehicleControlUpd/1 -> Sync_Out/1
  Demux2/2 -> Bus Creator2/2  "VhclCtrl BrakePark"
  Demux2/1 -> Bus Creator2/1  "VhclCtrl Brake"
